simulink model "sampleModel1538"  (R2023a)
settings: Solver=VariableStepAuto  StartTime=0.0  StopTime=10.0  RelTol=1e-3
libraries: hdlsllib x2, simulink x2
settings Model: Creator=user1  LastModifiedBy=user1

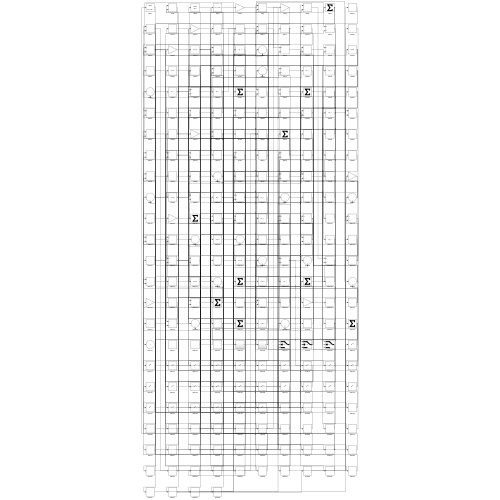
[thumbnail: Simulink's stored preview of the top-level diagram]
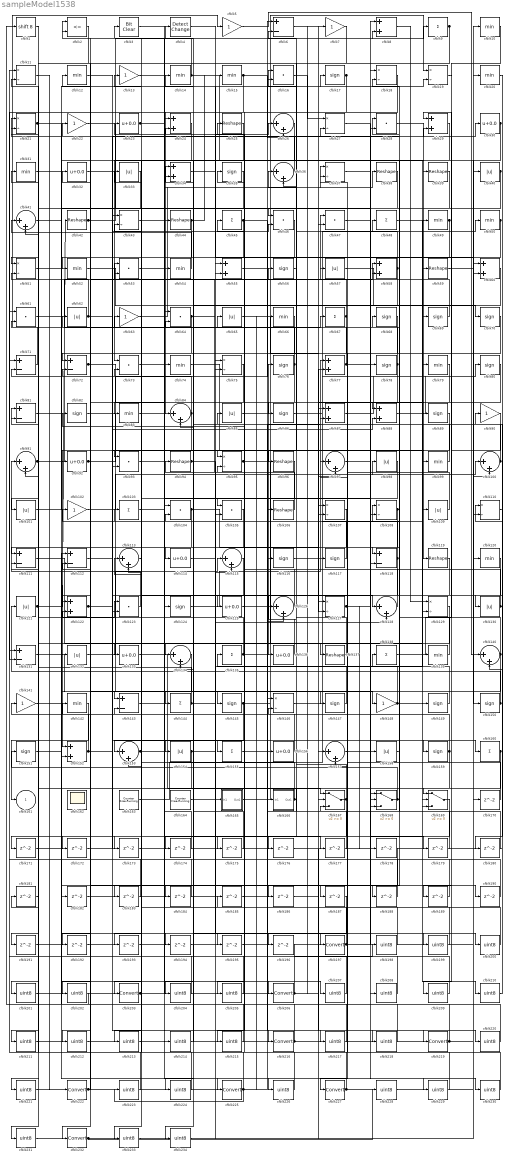
== system sampleModel1538 ==
  cfblk1 : ArithShift  BitShiftNumber=8
  cfblk{10,12,14..15,20,31,49..50,52,54,66,74,79,83,99,120,139,142} (18 alike) : MinMax
  cfblk{26,36,41,84,91,97,100,113,115,126,128,134,140,153,157} (15 alike) : Sum  Inputs=|++
  cfblk{33,40,57,62,65,85,98,101,109,121,130,132,154,158} (14 alike) : Abs  SaturateOnIntegerOverflow=off
  cfblk{5,7,13,22,63,90,102,141,148} (9 alike) : Gain
  cfblk{9,45,48,67,103,135,138,144,155,160} (10 alike) : Sum  Inputs=+
  cfblk{16,28,46..47,53,61,64,73,93,104..105,123} (12 alike) : DotProduct  OutDataTypeStr=Inherit: Inherit via internal rule
  cfblk{25,38..39,42,44,59,94,96,106,119,137} (11 alike) : Reshape
  cfblk{11,18..19,21,27,37,43,51,75,95,107..108,110,127,129,146} (16 alike) : Product  Inputs=*/  RndMeth=Zero  SaturateOnIntegerOverflow=on
  cfblk{6,71..72,81,111..112,118,131,143} (9 alike) : Sum  Inputs=+-
  cfblk{23,30,32,92,114,125,133,136,156} (9 alike) : Bias  Bias=0.0  SaturateOnIntegerOverflow=off
  cfblk{17,35,56,68..70,76,78,80,82,86,89,116..117,124,145,147,149..151,159} (21 alike) : Signum
  cfblk{8,24,29,34,55,58,60,77,87..88,122,152} (12 alike) : Sum
  cfblk162 : Scope
      settings: Floating=on
  cfblk163 : hdlsllib/Sources/Counter Free-Running  NumBits=16  tsamp=-1
  cfblk164 : hdlsllib/Sources/Counter Free-Running  NumBits=16  tsamp=-1
  cfblk165 : Subsystem
      settings: LibrarySourceBlock=|
      | hdlsllib/Ports &
      | Subsystems/Subsystem
  cfblk166 : Subsystem
      settings: LibrarySourceBlock=|
      | hdlsllib/Ports &
      | Subsystems/Subsystem
  cfblk167 : Switch  SaturateOnIntegerOverflow=off  InputSameDT=off
  cfblk168 : Switch  SaturateOnIntegerOverflow=off  InputSameDT=off
  cfblk169 : Switch  SaturateOnIntegerOverflow=off  InputSameDT=off
  cfblk{170..196} (27 alike) : Delay  SampleTime=1
  cfblk{197,203,206,216,219,222,225,227,232} (9 alike) : DataTypeConversion  SaturateOnIntegerOverflow=off  RndMeth=Floor
  cfblk{198..202,204..205,207..215,217..218,220..221,223..224,226,228..231,233..234} (29 alike) : DataTypeConversion  OutDataTypeStr=uint8  SaturateOnIntegerOverflow=off  RndMeth=Floor
  cfblk2 : RelationalOperator  Operator=<=  OutDataTypeStr=boolean  InputSameDT=off
  cfblk3 : simulink/Logic and Bit Operations/Bit Clear  iBit=0
      settings: LibrarySourceBlock=|
      | hdlsllib/Logic and Bit
      | Operations/Bit Clear
  cfblk4 : simulink/Logic and Bit Operations/Detect Change  vinit=0  OutDataTypeStr=boolean
      settings: LibrarySourceBlock=|
      | hdlsllib/Logic and Bit
      | Operations/Detect
      | Change
  cfblk161 : Outport  VectorParamsAs1DForOutWhenUnconnected=off
  wires:
  cfblk8/1 -> cfblk129/1
  cfblk132/1 -> cfblk115/1
  cfblk84/1 -> cfblk152/1, cfblk71/2
  cfblk120/1 -> cfblk227/1
  cfblk85/1 -> cfblk19/1
  cfblk28/1 -> cfblk119/1
  cfblk138/1 -> cfblk29/1
  cfblk56/1 -> cfblk95/1
  cfblk61/1 -> cfblk206/1
  cfblk148/1 -> cfblk56/1, cfblk210/1
  cfblk165/1(Out1) -> cfblk47/1
  cfblk5/1 -> cfblk140/1
  cfblk149/1 -> cfblk35/1
  cfblk121/1 -> cfblk42/1, cfblk190/1
  cfblk147/1 -> cfblk135/1
  cfblk16/1 -> cfblk27/1
  cfblk42/1 -> cfblk9/1, cfblk96/1
  cfblk18/1 -> cfblk84/1
  cfblk163/1 -> cfblk48/1
  cfblk33/1 -> cfblk52/1
  cfblk156/1 -> cfblk81/1
  cfblk131/1 -> cfblk148/1
  cfblk32/1 -> cfblk47/2
  cfblk168/1 -> cfblk58/1, cfblk151/1
  cfblk30/1 -> cfblk73/1, cfblk118/1, cfblk110/2
  cfblk81/1 -> cfblk65/1
  cfblk140/1 -> cfblk28/1, cfblk21/2, cfblk224/1
  cfblk36/1 -> cfblk22/1
  cfblk124/1 -> cfblk77/1
  cfblk119/1 -> cfblk136/1
  cfblk48/1 -> cfblk109/1
  cfblk88/1 -> cfblk80/1
  cfblk125/1 -> cfblk156/1
  cfblk82/1 -> cfblk145/1
  cfblk71/1 -> cfblk5/1
  cfblk19/1 -> cfblk169/1
  cfblk23/1 -> cfblk8/2, cfblk127/2, cfblk177/1
  cfblk58/1 -> cfblk36/2, cfblk184/1
  cfblk69/1 -> cfblk12/1
  cfblk126/1 -> cfblk102/1
  cfblk127/1 -> cfblk178/1, cfblk179/1
  cfblk136/1 -> cfblk76/1
  cfblk95/1 -> cfblk169/2, cfblk215/1
  cfblk133/1 -> cfblk167/1
  cfblk10/1 -> cfblk79/1
  cfblk94/1 -> cfblk165/1(In1), cfblk196/1
  cfblk60/1 -> cfblk144/1
  cfblk14/1 -> cfblk149/1, cfblk2/1
  cfblk116/1 -> cfblk8/1
  cfblk141/1 -> cfblk225/1
  cfblk158/1 -> cfblk68/1
  cfblk145/1 -> cfblk49/1, cfblk153/2
  cfblk80/1 -> cfblk154/1
  cfblk91/1 -> cfblk53/1, cfblk186/1
  cfblk44/1 -> cfblk132/1, cfblk15/1
  cfblk22/1 -> cfblk78/1
  cfblk128/1 -> cfblk82/1
  cfblk142/1 -> cfblk161/1
  cfblk76/1 -> cfblk31/1, cfblk134/2
  cfblk153/1 -> cfblk98/1, cfblk67/1
  cfblk64/1 -> cfblk30/1, cfblk123/2
  cfblk146/1 -> cfblk59/1
  cfblk7/1 -> cfblk86/1
  cfblk101/1 -> cfblk19/2
  cfblk63/1 -> cfblk37/1
  cfblk130/1 -> cfblk23/1, cfblk110/1
  cfblk87/1 -> cfblk60/1
  cfblk37/1 -> cfblk18/1
  cfblk21/1 -> cfblk39/1, cfblk194/1, cfblk230/1
  cfblk74/1 -> cfblk139/1
  cfblk45/1 -> cfblk74/1, cfblk137/1, cfblk195/1
  cfblk114/1 -> cfblk26/1
  cfblk55/1 -> cfblk219/1
  cfblk99/1 -> cfblk34/1
  cfblk67/1 -> cfblk25/1, cfblk122/1
  cfblk159/1 -> cfblk146/2, cfblk175/1, cfblk176/1
  cfblk34/1 -> cfblk46/1
  cfblk118/1 -> cfblk125/1, cfblk62/1, cfblk106/1
  cfblk117/1 -> cfblk16/1
  cfblk123/1 -> cfblk91/1
  cfblk39/1 -> cfblk92/1
  cfblk3/1 -> cfblk197/1
  cfblk6/1 -> cfblk89/1
  cfblk66/1 -> cfblk152/2
  cfblk109/1 -> cfblk64/2
  cfblk102/1 -> cfblk100/1
  cfblk111/1 -> cfblk158/1
  cfblk11/1 -> cfblk222/1
  cfblk24/1 -> cfblk143/1
  cfblk139/1 -> cfblk108/1
  cfblk92/1 -> cfblk6/1, cfblk88/2
  cfblk167/1 -> cfblk126/1, cfblk231/1
  cfblk115/1 -> cfblk153/1
  cfblk73/1 -> cfblk38/1
  cfblk86/1 -> cfblk69/1
  cfblk54/1 -> cfblk41/1
  cfblk104/1 -> cfblk133/1, cfblk127/1
  cfblk83/1 -> cfblk108/2
  cfblk41/1 -> cfblk44/1
  cfblk12/1 -> cfblk159/1
  cfblk164/1 -> cfblk17/1
  cfblk113/1 -> cfblk203/1
  cfblk38/1 -> cfblk91/2
  cfblk155/1 -> cfblk87/2
  cfblk40/1 -> cfblk83/1, cfblk168/3, cfblk189/1
  cfblk135/1 -> cfblk166/1(In1), cfblk111/2
  cfblk57/1 -> cfblk150/1
  cfblk160/1 -> cfblk168/2, cfblk191/1
  cfblk9/1 -> cfblk72/1, cfblk101/1
  cfblk89/1 -> cfblk93/1
  cfblk20/1 -> cfblk130/1
  cfblk77/1 -> cfblk32/1, cfblk33/1, cfblk99/1
  cfblk49/1 -> cfblk114/1, cfblk93/2
  cfblk157/1 -> cfblk50/1
  cfblk2/1 -> cfblk111/1
  cfblk62/1 -> cfblk21/1, cfblk58/2, cfblk128/1
  cfblk144/1 -> cfblk27/2, cfblk51/2
  cfblk100/1 -> cfblk63/1, cfblk45/1
  cfblk68/1 -> cfblk157/2
  cfblk137/1 -> cfblk6/2
  cfblk29/1 -> cfblk169/3
  cfblk78/1 -> cfblk4/1, cfblk205/1
  cfblk17/1 -> cfblk155/1, cfblk131/2
  cfblk112/1 -> cfblk216/1
  cfblk4/1 -> cfblk60/2
  cfblk70/1 -> cfblk105/1
  cfblk108/1 -> cfblk187/1, cfblk188/1
  cfblk106/1 -> cfblk94/1
  cfblk150/1 -> cfblk121/1, cfblk85/1
  cfblk151/1 -> cfblk123/1
  cfblk50/1 -> cfblk129/2, cfblk88/1
  cfblk15/1 -> cfblk51/1, cfblk26/2
  cfblk65/1 -> cfblk117/1
  cfblk72/1 -> cfblk124/1, cfblk29/2
  cfblk154/1 -> cfblk138/1, cfblk128/2, cfblk221/1
  cfblk47/1 -> cfblk168/1
  cfblk122/1 -> cfblk57/1, cfblk160/1, cfblk134/1
  cfblk52/1 -> cfblk70/1
  cfblk152/1 -> cfblk46/2, cfblk142/1
  cfblk143/1 -> cfblk54/1
  cfblk59/1 -> cfblk20/1
  cfblk75/1 -> cfblk232/1
  cfblk166/1(Out1) -> cfblk43/2, cfblk16/2
  cfblk31/1 -> cfblk147/1
  cfblk170/1 -> cfblk37/2
  cfblk129/1 -> cfblk171/1
  cfblk171/1 -> cfblk140/2
  cfblk169/1 -> cfblk172/1
  cfblk172/1 -> cfblk43/1
  cfblk98/1 -> cfblk173/1
  cfblk173/1 -> cfblk115/2
  cfblk25/1 -> cfblk174/1
  cfblk174/1 -> cfblk24/1
  cfblk175/1 -> cfblk84/2
  cfblk177/1 -> cfblk36/1
  cfblk179/1 -> cfblk146/1
  cfblk110/1 -> cfblk180/1
  cfblk180/1 -> cfblk18/2
  cfblk181/1 -> cfblk41/2
  cfblk51/1 -> cfblk182/1
  cfblk182/1 -> cfblk77/2
  cfblk105/1 -> cfblk183/1
  cfblk183/1 -> cfblk71/1
  cfblk184/1 -> cfblk72/2
  cfblk188/1 -> cfblk167/3
  cfblk189/1 -> cfblk143/2
  cfblk190/1 -> cfblk2/2
  cfblk191/1 -> cfblk28/2
  cfblk134/1 -> cfblk192/1
  cfblk192/1 -> cfblk100/2
  cfblk26/1 -> cfblk193/1
  cfblk193/1 -> cfblk157/1
  cfblk194/1 -> cfblk167/2
  cfblk195/1 -> cfblk126/2
  cfblk197/1 -> cfblk118/2, cfblk64/1
  cfblk196/1 -> cfblk198/1
  cfblk198/1 -> cfblk3/1
  cfblk185/1 -> cfblk199/1
  cfblk199/1 -> cfblk104/2
  cfblk53/1 -> cfblk200/1
  cfblk200/1 -> cfblk185/1
  cfblk1/1 -> cfblk201/1
  cfblk201/1 -> cfblk104/1
  cfblk178/1 -> cfblk202/1
  cfblk202/1 -> cfblk1/1
  cfblk203/1 -> cfblk105/2, cfblk87/1
  cfblk79/1 -> cfblk204/1
  cfblk204/1 -> cfblk113/1
  cfblk205/1 -> cfblk113/2
  cfblk206/1 -> cfblk181/1, cfblk7/1
  cfblk13/1 -> cfblk207/1
  cfblk207/1 -> cfblk61/1
  cfblk27/1 -> cfblk208/1
  cfblk208/1 -> cfblk61/2
  cfblk90/1 -> cfblk209/1
  cfblk209/1 -> cfblk81/2
  cfblk210/1 -> cfblk90/1
  cfblk107/1 -> cfblk211/1
  cfblk211/1 -> cfblk170/1
  cfblk46/1 -> cfblk212/1
  cfblk212/1 -> cfblk107/1
  cfblk35/1 -> cfblk213/1
  cfblk213/1 -> cfblk107/2
  cfblk103/1 -> cfblk214/1
  cfblk214/1 -> cfblk34/2
  cfblk215/1 -> cfblk103/1
  cfblk216/1 -> cfblk131/1, cfblk14/1
  cfblk43/1 -> cfblk217/1
  cfblk217/1 -> cfblk112/1
  cfblk176/1 -> cfblk218/1
  cfblk218/1 -> cfblk112/2
  cfblk219/1 -> cfblk73/2, cfblk24/2
  cfblk186/1 -> cfblk220/1
  cfblk220/1 -> cfblk55/1
  cfblk221/1 -> cfblk55/2
  cfblk222/1 -> cfblk122/2, cfblk116/1
  cfblk223/1 -> cfblk11/1
  cfblk224/1 -> cfblk11/2
  cfblk225/1 -> cfblk223/1, cfblk66/1, cfblk13/1
  cfblk93/1 -> cfblk226/1
  cfblk226/1 -> cfblk141/1
  cfblk227/1 -> cfblk53/2, cfblk10/1
  cfblk228/1 -> cfblk120/1
  cfblk97/1 -> cfblk229/1
  cfblk229/1 -> cfblk95/2
  cfblk230/1 -> cfblk97/1
  cfblk231/1 -> cfblk97/2
  cfblk232/1 -> cfblk228/1, cfblk40/1
  cfblk96/1 -> cfblk233/1
  cfblk233/1 -> cfblk75/1
  cfblk187/1 -> cfblk234/1
  cfblk234/1 -> cfblk75/2

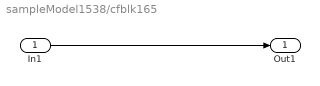
== system sampleModel1538/cfblk165 ==
  In1 : Inport
  Out1 : Outport
  wires:
  In1/1 -> Out1/1

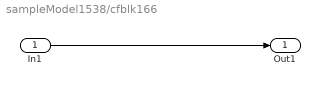
== system sampleModel1538/cfblk166 ==
  In1 : Inport
  Out1 : Outport
  wires:
  In1/1 -> Out1/1
